simulink model "VOO"  (R2022a)
settings: Solver=FixedStepAuto  StartTime=0.0  StopTime=10.0  FixedStep=1e-3  RelTol=1e-3  EnableMultiTasking=on
undefined symbols (not defined in the file): D10, D11, D2, D4, D5, D8, PTA0, PTA2, PTB23, PTB9, PTD0, PTD2
libraries: frdmk64flib x6
settings Model: ExtModeTrigDuration=5  Creator=bgdiv  LastModifiedBy=bgdiv
settings OptimizationCC: EnhancedBackFolding=on  PassReuseOutputArgsAs=Individual arguments  ZeroExternalMemoryAtStartup=off  ZeroInternalMemoryAtStartup=off  MaxStackSize=64  OptimizeBlockOrder=speed  DifferentSizesBufferReuse=on  OptimizationCustomize=off  EfficientTunableParamExpr=on
settings DebuggingCC: ParameterTunabilityLossMsg=error
settings HardwareCC: ProdBitPerPointer=32  ProdBitPerSizeT=32  ProdBitPerPtrDiffT=32  ProdLargestAtomicInteger=Long  ProdLargestAtomicFloat=Double  ProdWordSize=32  ProdHWDeviceType=ARM Compatible->ARM Cortex
settings SFSimCC: MATLABDynamicMemAlloc=off
settings RTWCC: SystemTargetFile=ert.tlc  HardwareBoard=NXP FRDM-K64F  TLCOptions="-aInlineSetEventsForThisBaseRateFcn=TLC_FALSE -aSuppressMultiTaskScheduler=TLC_FALSE  -aRateBasedStepFcn=0"  TemplateMakefile=ert_default_tmf  Toolchain=GNU Tools for ARM Embedded Processors
settings CodeAppCC: ForceParamTrailComments=on  IgnoreCustomStorageClasses=off  OperatorAnnotations=on  SimulinkDataObjDesc=on  SFDataObjDesc=on  InsertBlockDesc=on
settings ERTTargetCC: ExtModeTransport=4  ExtModeMexFile=sendToCommService

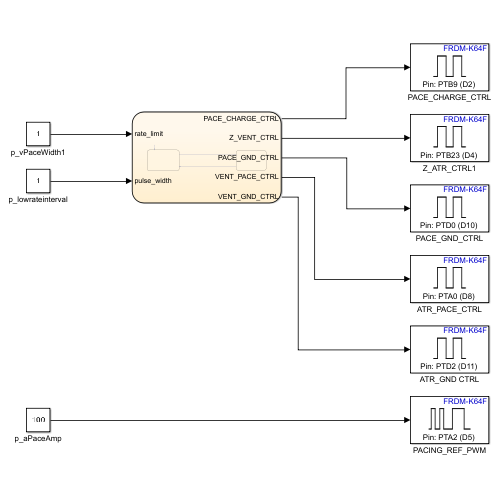
[thumbnail: Simulink's stored preview of the top-level diagram]
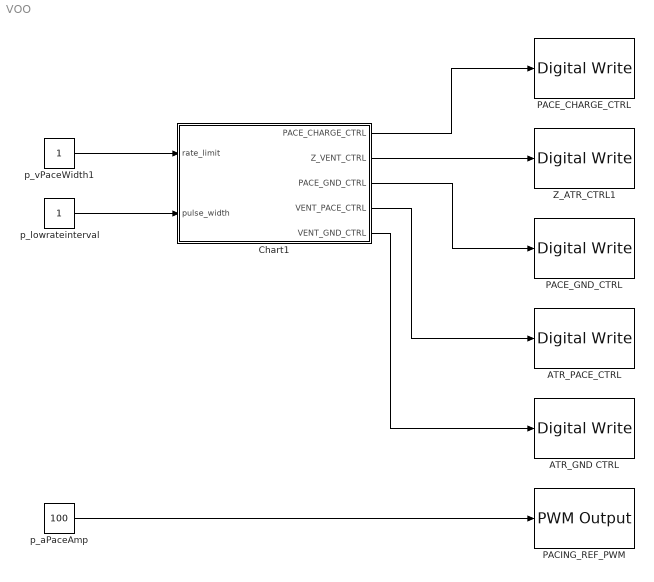
== system VOO ==
  ATR_GND CTRL : frdmk64flib/Digital Write  Whichpin=PTD2 (D11)
  ATR_PACE_CTRL : frdmk64flib/Digital Write  Whichpin=PTA0 (D8)
  Chart1 : Stateflow chart  TreatAsAtomicUnit=on
  PACE_CHARGE_CTRL : frdmk64flib/Digital Write  Whichpin=PTB9 (D2)
  PACE_GND_CTRL : frdmk64flib/Digital Write  Whichpin=PTD0 (D10)
  PACING_REF_PWM : frdmk64flib/PWM Output  Whichpin=PTA2 (D5)  InitialFrequency=2000  InitialDutyCycle=0
  Z_ATR_CTRL1 : frdmk64flib/Digital Write  Whichpin=PTB23 (D4)
  p_aPaceAmp : Constant  Value=100
  p_lowrateinterval : Constant
  p_vPaceWidth1 : Constant
  wires:
  p_lowrateinterval/1 -> Chart1/2(pulse_width)
  p_vPaceWidth1/1 -> Chart1/1(rate_limit)
  p_aPaceAmp/1 -> PACING_REF_PWM/1
  Chart1/1(PACE_CHARGE_CTRL) -> PACE_CHARGE_CTRL/1
  Chart1/2(Z_VENT_CTRL) -> Z_ATR_CTRL1/1
  Chart1/3(PACE_GND_CTRL) -> PACE_GND_CTRL/1
  Chart1/4(VENT_PACE_CTRL) -> ATR_PACE_CTRL/1
  Chart1/5(VENT_GND_CTRL) -> ATR_GND CTRL/1

== stateflow chart VOO/Chart1 ==
  state Charging_Discharging
    entry:
    VENT_PACE_CTRL = false
    PACE_CHARGE_CTRL = true
    VENT_GND_CTRL = true
    PACE_GND_CTRL = true
    Z_VENT_CTRL=false
  state Pace_Heart
    entry:
    VENT_PACE_CTRL = true
    PACE_CHARGE_CTRL = false
    PACE_GND_CTRL = true
    VENT_GND_CTRL = false
  (default) -> Charging_Discharging
  Charging_Discharging -> Pace_Heart : after(((1/rate_limit)*60000)-pulse_width,msec)
  Pace_Heart -> Charging_Discharging : after(pulse_width,msec)
  data: rate_limit input; pulse_width input; PACE_CHARGE_CTRL output boolean; Z_VENT_CTRL output boolean; PACE_GND_CTRL output boolean; VENT_PACE_CTRL output boolean; VENT_GND_CTRL output boolean
